simulink model "test_01"  (R2022b)
settings: Solver=VariableStepAuto  StartTime=0.0  StopTime=5  RelTol=1e-3
values from neighbouring files (symbols this model uses):
  C = Vout*(1-d/100)/(8*dV*f*f*L)    (= 6.25e-05)    [params.m]
  L = Vout*(1-d/100)/(f*dI)    (= 0.00990566037736)    [params.m]
undefined symbols (not defined in the file or in its folder): Ion, Lithium
libraries: spsThyristorLib x6, spsSeriesRLCBranchLib x3, spsVoltageMeasurementLib x3, spsCurrentMeasurementLib x2, spsGroundLib x1, spsThreePhaseProgrammableVoltageSourceLib x1, spsThreePhaseVIMeasurementLib x1, spsBatteryLib x1, spsDiodeLib x1, spsIGBTDiodeLib x1, slpidlib x1, spsTriangleGeneratorLib x1
settings Model: Creator=sanke  LastModifiedBy=sanke
settings SolverCC: ZeroCrossAlgorithm=Adaptive
settings DebuggingCC: IgnoredZcDiagnostic=none

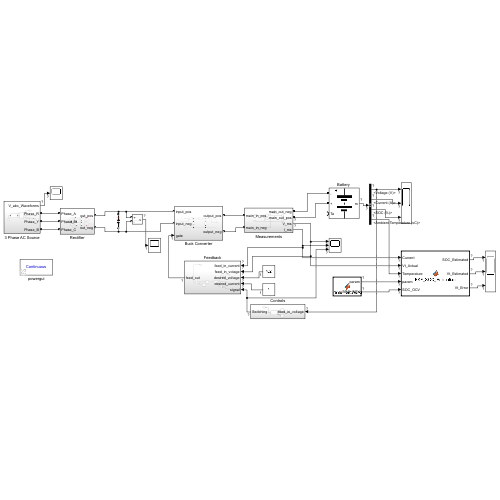
[thumbnail: Simulink's stored preview of the top-level diagram]
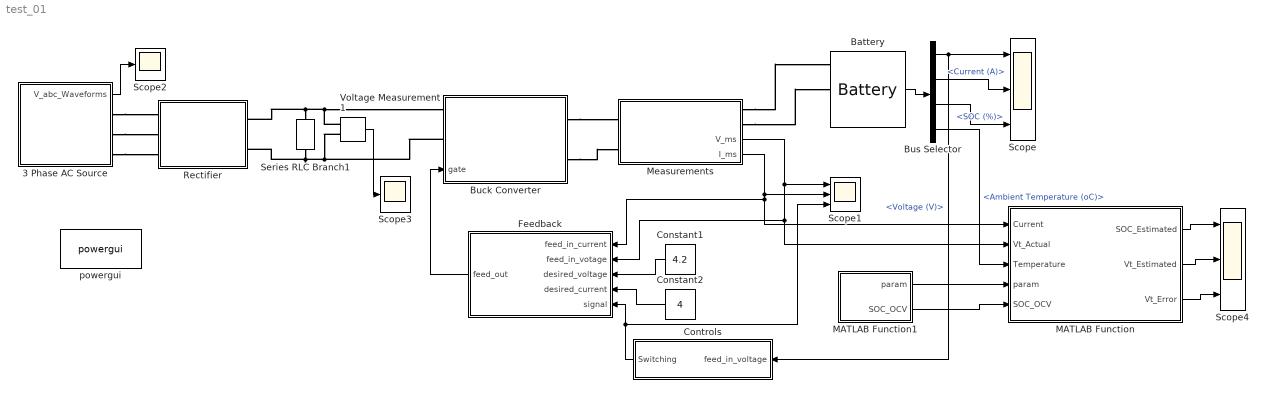
== system test_01 ==
  3 Phase AC Source : Subsystem
  "Battery " : spsBatteryLib/Battery  BatType=Lithium-Ion  ShowTempParam=on  ThermalPreset="3.6V  3.6Ah  (LiNiO2)"  ShowAgeParam=off  NomV=3.1  NomQ=3.6  SOC=55  Batt_Tr=30  PresetModel=off  MaxQ=3.2  MinV=2.325  FullV=3.75  Dis_rate=0.72  R=0.00889  Normal_OP=2.8  expZone="[3.5         0.5]"  current=[6.5 13 32.5]  Units=Time  Tci=20  NomT=20  T2=0  MaxQ2=2.7  FullV2=3.5  Normal_OP2=2.94  expZone2="[3.25         0.5]"  Rca=0.6  ti=1000  Dp=0  Neq0=0  Tsim=1e6  Ta1=25  Qeol=5.4*0.9  Reol=0.013333*1.2  Char_age=[2.3478, 3]  Dis_age=[2.3478, 10]  N1=1500  N2=10500  N3=1000  N4=1400  Ta2=45  N5=950
  Buck Converter : Subsystem
      settings: PortSchema="{\"entries\":[{\"content\":{\"sides\":[{\"content\":{\"connectorIds\":[\"LConn1\",\"LConn2\",\"In1\"]},\"type\":\"ConnectorPlacement.EquallySpacedRectSide\",\"uuid\":\"8046495b-0d90-4cb8-9891-48dc7aace6d4\"},{\"content\":{\"connectorIds\":[\"RConn1\",\"RConn2\"],\"side\":\"RIGHT\"},\"type\":\"ConnectorPlacement.EquallySpacedRectSide\",\"uuid\":\"421d384b-a39e-4e59-844e-5fb42b3432e4\"},{\"content\":{\"connectorIds\":[],\"side\":\"TOP\"},\"type\":\"ConnectorPlacement.EquallySpacedRectSide\",\"uuid\":\"a93954f5-8cef-4771-909c-d15532f662fe\"}]},\"type\":\"ConnectorPlacement.EquallySpacedConnector\",\"uuid\":\"185038a6-0d13-426c-9082-f1ae7959dda3\"}],\"packageUris\":[\"http://schema.mathworks.com/mf0/Connector/R2020b\"],\"version\":\"1.0\"}"
  Bus Selector : BusSelector  OutputSignals=Voltage (V),Current (A),SOC (%),Ambient Temperature (oC)
  Constant1 : Constant  Value=4.2
  Constant2 : Constant  Value=4
  Controls : Subsystem
  Feedback : Subsystem
  MATLAB Function : MATLAB Function  TreatAsAtomicUnit=on
  MATLAB Function1 : MATLAB Function  TreatAsAtomicUnit=on
  Measurements : Subsystem
      settings: PortSchema="{\"entries\":[{\"content\":{\"sides\":[{\"content\":{\"connectorIds\":[\"LConn1\",\"LConn2\"]},\"type\":\"ConnectorPlacement.EquallySpacedRectSide\",\"uuid\":\"fbcba962-5f19-4ca0-9e90-c21659520055\"},{\"content\":{\"connectorIds\":[\"RConn1\",\"RConn2\",\"Out1\",\"Out2\"],\"side\":\"RIGHT\"},\"type\":\"ConnectorPlacement.EquallySpacedRectSide\",\"uuid\":\"9e6fe38e-ff6b-4271-81f9-afd15cda60bb\"},{\"content\":{\"connectorIds\":[],\"side\":\"TOP\"},\"type\":\"ConnectorPlacement.EquallySpacedRectSide\",\"uuid\":\"0e1fc647-5705-4062-8d37-f05674e3ac40\"}]},\"type\":\"ConnectorPlacement.EquallySpacedConnector\",\"uuid\":\"9c5396ba-9d04-4277-89c0-94d7fbac7837\"}],\"packageUris\":[\"http://schema.mathworks.com/mf0/Connector/R2020b\"],\"version\":\"1.0\"}"
  Rectifier : Subsystem
  Scope : Scope  NumInputPorts=3
  Scope1 : Scope  NumInputPorts=3
  Scope2 : Scope
  Scope3 : Scope
  Scope4 : Scope  NumInputPorts=3
  Series RLC Branch1 : spsSeriesRLCBranchLib/Series RLC Branch  LConnTagsString=__new0  RConnTagsString=__new0  BranchType=C  Resistance=1  Inductance=1e-3  SetiL0=off  InitialCurrent=0  Capacitance=1000e-6  Setx0=off  InitialVoltage=0  Measurements=None
  Voltage Measurement1 : spsVoltageMeasurementLib/Voltage Measurement  PhasorSimulation=off  OutputType=Complex  PSBequivalent=0
  powergui : sps_lib/powergui  Priority=1  SimulationMode=Continuous  SampleTime=0.01  frequency=60  Iterations=50  frequencyindice=0  Pbase=100e6  ErrMax=1e-4  UnitsV=kV  UnitsW=MW  buscounter=0  FunctionMessages=off  echomessages=off  EnableUseOfTLC=off  CurrentSourceSwitches=off  DisableSnubberDevices=off  DisableRonSwitches=off  DisableVfSwitches=off  DisplayEquations=off  AutomaticDiscreteSolvers=off  SolverType=Tustin/Backward Euler (TBE)  Interpol=off  ExternalGateDelay=off  methode=off  Ts=100  x0status=blocks  SPID=on  SwTol=0  HookPort=off  NonlinearTolerance=1e-4  nMaxIteration=100  ContinueOnMaxIteration=off  RestoreLinks=warning  ResistiveCurrentMeasurement=off  Frange=[0:2:500]  Ylog=off  Xlog=on  ShowGrid=off  save=off  variable=ZData  structure=0  ZoomFFT=off  StartTime=0.0  cycles=1  DisplayStyle=1  fundamental=60  FreqAxis=off  MaxFrequency=1000  frequencyindicesteady=1  RmsSteady=1  display=off
  wires:
  Voltage Measurement1/1 -> Scope3/1
  3 Phase AC Source/1(V_abc_Waveforms) -> Scope2/1
  Constant1/1 -> Feedback/3(desired_voltage)
  Feedback/1(feed_out) -> Buck Converter/1(gate)
  Measurements/1(V_ms) -> MATLAB Function/2(Vt_Actual), Feedback/2(feed_in_votage), Scope1/1
  Measurements/2(I_ms) -> MATLAB Function/1(Current), Feedback/1(feed_in_current), Scope1/2
  Constant2/1 -> Feedback/4(desired_current)
  Controls/1(Switching) -> Scope1/3, Feedback/5(signal)
  "Battery "/1 -> Bus Selector/1
  Bus Selector/2 -> Scope/2  "<Current (A)>"
  Bus Selector/1 -> Controls/1(feed_in_voltage), Scope/1  "<Voltage (V)>"
  Bus Selector/3 -> Scope/3  "<SOC (%)>"
  Bus Selector/4 -> MATLAB Function/3(Temperature)  "<Ambient Temperature (oC)>"
  MATLAB Function/1(SOC_Estimated) -> Scope4/1
  MATLAB Function/2(Vt_Estimated) -> Scope4/2
  MATLAB Function/3(Vt_Error) -> Scope4/3
  MATLAB Function1/1(param) -> MATLAB Function/4(param)
  MATLAB Function1/2(SOC_OCV) -> MATLAB Function/5(SOC_OCV)
  connections:
  Voltage Measurement1/LConn1 -- Series RLC Branch1/LConn1 -- Rectifier/RConn1 -- Buck Converter/LConn1
  Voltage Measurement1/LConn2 -- Series RLC Branch1/RConn1 -- Rectifier/RConn2 -- Buck Converter/LConn2
  3 Phase AC Source/RConn1 -- Rectifier/LConn1
  3 Phase AC Source/RConn3 -- Rectifier/LConn3
  3 Phase AC Source/RConn2 -- Rectifier/LConn2
  Buck Converter/RConn2 -- Measurements/LConn2
  Buck Converter/RConn1 -- Measurements/LConn1
  Measurements/RConn1 -- "Battery "/LConn2
  Measurements/RConn2 -- "Battery "/LConn1

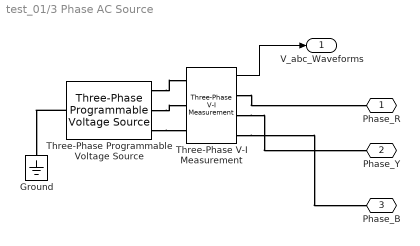
== system test_01/3 Phase AC Source ==
  Ground : spsGroundLib/Ground  LConnTagsString=a
  Three-Phase Programmable Voltage Source : spsThreePhaseProgrammableVoltageSourceLib/Three-Phase Programmable Voltage Source  PositiveSequence="[230*sqrt(2)  0 50]"  VariationEntity=None  VariationType=Table of time-amplitude pairs  VariationTypeAlt=Step  VariationStep=0.5  VariationRate=10  VariationMagnitude=0.3  VariationFrequency=2  VariationTiming=[1 2]  VariationPhaseA=off  Amplitudes=[1 0.8 1.2 1.0]  TimeValues=[0 0.1 0.15 0.2]  HarmonicGeneration=off  HarmonicA=[3 0.2 -25 0]  HarmonicB=[2 0.15 35 2]  Timing="[0.05  3]"  BusType=swing  Pref=0  Qref=0  Qmin=-inf  Qmax=inf
  Three-Phase V-I Measurement : spsThreePhaseVIMeasurementLib/Three-Phase V-I Measurement  VoltageMeasurement=phase-to-ground  SetLabelV=off  LabelV=Vabc  Vpu=off  VpuLL=off  CurrentMeasurement=no  SetLabelI=off  LabelI=Iabc  Ipu=off  Pbase=100e6  Vbase=500e3  OutputType=Complex  PhasorSimulation=off  PSBequivalent=0
  Phase_R : PMIOPort  Side=Right
  Phase_Y : PMIOPort  Port=2  Side=Right
  Phase_B : PMIOPort  Port=3  Side=Right
  V_abc_Waveforms : Outport
  wires:
  Three-Phase V-I Measurement/1 -> V_abc_Waveforms/1
  connections:
  Three-Phase Programmable Voltage Source/RConn1 -- Three-Phase V-I Measurement/LConn1
  Three-Phase Programmable Voltage Source/LConn1 -- Ground/LConn1
  Three-Phase Programmable Voltage Source/RConn2 -- Three-Phase V-I Measurement/LConn2
  Three-Phase Programmable Voltage Source/RConn3 -- Three-Phase V-I Measurement/LConn3
  Three-Phase V-I Measurement/RConn1 -- Phase_R/RConn1
  Three-Phase V-I Measurement/RConn2 -- Phase_Y/RConn1
  Three-Phase V-I Measurement/RConn3 -- Phase_B/RConn1

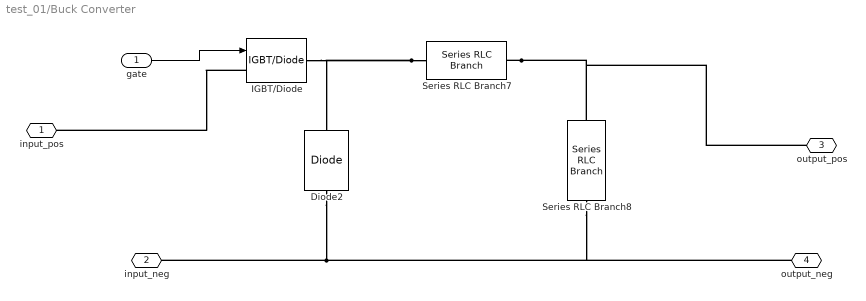
== system test_01/Buck Converter ==
  gate : Inport
  Diode2 : spsDiodeLib/Diode  Ron=0.001  Lon=0  Vf=0  IC=0  UseSnubber=0  Rs=500  Cs=250e-9  Measurements=off
  IGBT/Diode : spsIGBTDiodeLib/IGBT//Diode  Ron=1e-3  Rs=1e5  Cs=inf  Measurements=off
  Series RLC Branch7 : spsSeriesRLCBranchLib/Series RLC Branch  LConnTagsString=__new0  RConnTagsString=__new0  BranchType=L  Resistance=1  Inductance=L  SetiL0=off  InitialCurrent=0  Capacitance=1e-6  Setx0=off  InitialVoltage=0  Measurements=None
  Series RLC Branch8 : spsSeriesRLCBranchLib/Series RLC Branch  LConnTagsString=__new0  RConnTagsString=__new0  BranchType=C  Resistance=1  Inductance=1e-3  SetiL0=off  InitialCurrent=0  Capacitance=C  Setx0=off  InitialVoltage=0  Measurements=None
  input_pos : PMIOPort  Side=Left
  input_neg : PMIOPort  Port=2  Side=Left
  output_pos : PMIOPort  Port=3  Side=Right
  output_neg : PMIOPort  Port=4  Side=Right
  wires:
  gate/1 -> IGBT/Diode/1
  connections:
  IGBT/Diode/LConn1 -- input_pos/RConn1
  Series RLC Branch7/LConn1 -- IGBT/Diode/RConn1 -- Diode2/RConn1
  Series RLC Branch7/RConn1 -- output_pos/RConn1 -- Series RLC Branch8/LConn1
  Diode2/LConn1 -- Series RLC Branch8/RConn1 -- output_neg/RConn1 -- input_neg/RConn1

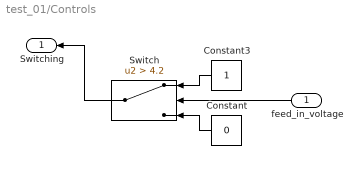
== system test_01/Controls ==
  feed_in_voltage : Inport
  Constant : Constant  Value=0
  Constant3 : Constant
  Switch : Switch  Criteria=u2 > Threshold  Threshold=4.2  SaturateOnIntegerOverflow=off  InputSameDT=off
  Switching : Outport
  wires:
  feed_in_voltage/1 -> Switch/2
  Switch/1 -> Switching/1
  Constant3/1 -> Switch/1
  Constant/1 -> Switch/3

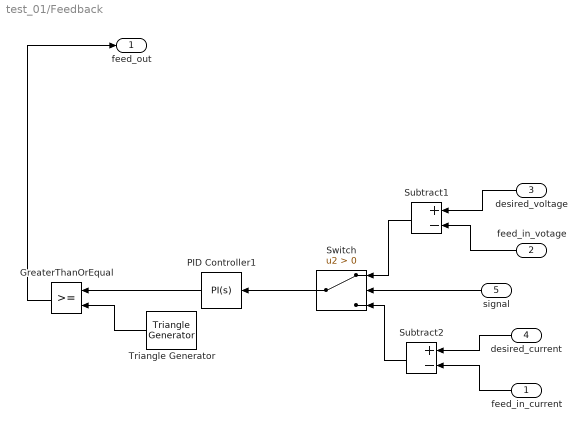
== system test_01/Feedback ==
  feed_in_current : Inport
  feed_in_votage : Inport  Port=2
  desired_voltage : Inport  Port=3
  desired_current : Inport  Port=4
  signal : Inport  Port=5
  GreaterThanOrEqual : RelationalOperator  OutDataTypeStr=boolean  RndMeth=Simplest  InputSameDT=off
  PID Controller1 : slpidlib/PID Controller  Controller=PI  Form=Parallel  TimeDomain=Continuous-time  UseExternalTs=off  SampleTime=-1  IntegratorMethod=Forward Euler  FilterMethod=Forward Euler  ControllerParametersSource=internal  P=50  I=5  UseKiTs=off  D=0  N=100  UseFilter=on  TunerSelectOption=Transfer Function Based (PID Tuner App)  InitialConditionSource=internal  InitialConditionForIntegrator=0  InitialConditionForFilter=0  DifferentiatorICPrevScaledInput=0  ExternalReset=none  TrackingMode=off  Kt=1  LimitOutput=off  SatLimitsSource=internal  UpperSaturationLimit=inf  LowerSaturationLimit=-inf  LinearizeAsGain=on  AntiWindupMode=none  Kb=1  LimitIntegrator=off  UpperIntegratorSaturationLimit=inf  LowerIntegratorSaturationLimit=-inf  POutMin=[]  POutMax=[]  IOutMin=[]  IOutMax=[]  DOutMin=[]  DOutMax=[]  NOutMin=[]  NOutMax=[]  SumOutMin=[]  SumOutMax=[]  SaturationOutMin=[]  SaturationOutMax=[]  PParamMin=[]  PParamMax=[]  IParamMin=[]  IParamMax=[]  DParamMin=[]  DParamMax=[]  NParamMin=[]  NParamMax=[]  KbParamMin=[]  KbParamMax=[]  KtParamMin=[]  KtParamMax=[]  KbOutMin=[]  KbOutMax=[]  KtOutMin=[]  KtOutMax=[]  IntegratorOutMin=[]  IntegratorOutMax=[]  FilterOutMin=[]  FilterOutMax=[]  SumI1OutMin=[]  SumI1OutMax=[]  SumI2OutMin=[]  SumI2OutMax=[]  SumI3OutMin=[]  SumI3OutMax=[]  SumI4OutMin=[]  SumI4OutMax=[]  SumDOutMin=[]  SumDOutMax=[]  DifferentiatorOutMin=[]  DifferentiatorOutMax=[]  FilterDiffOutCoefMin=[]  FilterDiffOutCoefMax=[]  ReciprocalOutMin=[]  ReciprocalOutMax=[]  SumDenOutMin=[]  SumDenOutMax=[]  SumNumOutMin=[]  SumNumOutMax=[]  DivideOutMin=[]  DivideOutMax=[]  UdiffTsProdOutMin=[]  UdiffTsProdOutMax=[]  NTsProdOutMin=[]  NTsProdOutMax=[]  UintegralTsProdOutMin=[]  UintegralTsProdOutMax=[]  UngainTsProdOutMin=[]  UngainTsProdOutMax=[]  ClampingZeroOutDataTypeStr=Inherit: Inherit via back propagation  ClampingZeroOutMin=[]  ClampingZeroOutMax=[]  FilterDenConstantOutDataTypeStr=Inherit: Inherit via back propagation  FilterDenConstantOutMin=[]  FilterDenConstantOutMax=[]  PCopyOutDataTypeStr=Inherit: Inherit via back propagation  PCopyOutMin=[]  PCopyOutMax=[]  NCopyOutDataTypeStr=Inherit: Inherit via back propagation  NCopyOutMin=[]  NCopyOutMax=[]  IntegratorContinuousStateAttributes=''  IntegratorStateMustResolveToSignalObject=off  IntegratorRTWStateStorageClass=Auto  FilterContinuousStateAttributes=''  FilterStateMustResolveToSignalObject=off  FilterRTWStateStorageClass=Auto  ParallelPVariant=InternalParameters  IdealPVariant=Disabled  IVariant=InternalParameters  DVariant=Disabled  IntegratorVariant=Continuous  SatVariant=Disabled  AWVariant=Passthrough  PCopyVariant=Disabled  TRVariant=Disabled  FdbkBlocksVariant=Forward  IdealPFdbkVariant=Disabled  SatFdbkVariant=Disabled  DerivativeFilterVariant=Disabled  NVariant=Disabled  NCopyVariant=Disabled_SignalSpec  FilterICVariant=Disabled  IntegratorICVariant=InternalICs  ExternalResetVariant=Disabled  TRSumVariant=Passthrough  SumFdbkVariant=Disabled  SumVariant=Sum_PI  TsampFilterVariant=InternalTs  TsampNgainVariant=Passthrough  TsampIntegralVariant=Passthrough  ExternalSaturationOutDataTypeStr=Inherit: Same as second input
  Subtract1 : Sum  Inputs=+-
  Subtract2 : Sum  Inputs=+-
  Switch : Switch  Criteria=u2 > Threshold  SaturateOnIntegerOverflow=off  InputSameDT=off
  Triangle Generator : spsTriangleGeneratorLib/Triangle Generator  Freq=25e3  Phase=90  Ts=0
  feed_out : Outport
  wires:
  Triangle Generator/1 -> GreaterThanOrEqual/2
  GreaterThanOrEqual/1 -> feed_out/1
  PID Controller1/1 -> GreaterThanOrEqual/1
  signal/1 -> Switch/2
  Subtract2/1 -> Switch/3
  desired_current/1 -> Subtract2/1
  feed_in_current/1 -> Subtract2/2
  desired_voltage/1 -> Subtract1/1
  feed_in_votage/1 -> Subtract1/2
  Subtract1/1 -> Switch/1
  Switch/1 -> PID Controller1/1

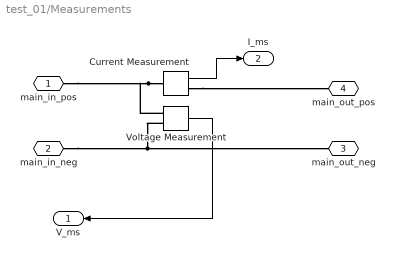
== system test_01/Measurements ==
  Current Measurement : spsCurrentMeasurementLib/Current Measurement  PhasorSimulation=off  OutputType=Complex  PSBequivalent=0
  Voltage Measurement : spsVoltageMeasurementLib/Voltage Measurement  PhasorSimulation=off  OutputType=Complex  PSBequivalent=0
  main_in_pos : PMIOPort  Side=Left
  main_in_neg : PMIOPort  Port=2  Side=Left
  main_out_neg : PMIOPort  Port=3  Side=Right
  main_out_pos : PMIOPort  Port=4  Side=Right
  V_ms : Outport
  I_ms : Outport  Port=2
  wires:
  Voltage Measurement/1 -> V_ms/1
  Current Measurement/1 -> I_ms/1
  connections:
  Current Measurement/LConn1 -- main_in_pos/RConn1 -- Voltage Measurement/LConn1
  Current Measurement/RConn1 -- main_out_pos/RConn1
  Voltage Measurement/LConn2 -- main_out_neg/RConn1 -- main_in_neg/RConn1

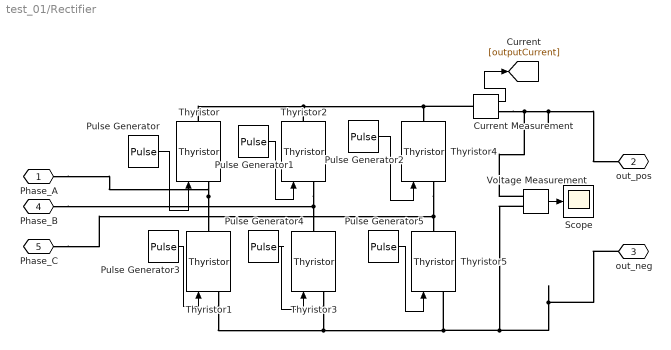
== system test_01/Rectifier ==
  Current Measurement : spsCurrentMeasurementLib/Current Measurement  PhasorSimulation=off  OutputType=Complex  PSBequivalent=0
  Pulse Generator : DiscretePulseGenerator  PulseType=Time based  Period=1/50  PulseWidth=33.33  PhaseDelay=(30+30)*0.02/360
  Pulse Generator1 : DiscretePulseGenerator  PulseType=Time based  Period=1/50  PulseWidth=33.33  PhaseDelay=(150+30)*0.02/360
  Pulse Generator2 : DiscretePulseGenerator  PulseType=Time based  Period=1/50  PulseWidth=33.33  PhaseDelay=(270+30)*0.02/360
  Pulse Generator3 : DiscretePulseGenerator  PulseType=Time based  Period=1/50  PulseWidth=33.33  PhaseDelay=(210+30)*0.02/360
  Pulse Generator4 : DiscretePulseGenerator  PulseType=Time based  Period=1/50  PulseWidth=33.33  PhaseDelay=(330+30)*0.02/360
  Pulse Generator5 : DiscretePulseGenerator  PulseType=Time based  Period=1/50  PulseWidth=33.33  PhaseDelay=(90+30)*0.02/360
  Scope : Scope
  Thyristor{,1..5} (6 alike) : spsThyristorLib/Thyristor  Ron=0.001  Lon=0  Vf=0.8  IC=0  Rs=500  Cs=250e-9  Measurements=off
  Voltage Measurement : spsVoltageMeasurementLib/Voltage Measurement  PhasorSimulation=off  OutputType=Complex  PSBequivalent=0
  Phase_A : PMIOPort  Side=Left
  out_pos : PMIOPort  Port=2  Side=Right
  out_neg : PMIOPort  Port=3  Side=Right
  Phase_B : PMIOPort  Port=4  Side=Left
  Phase_C : PMIOPort  Port=5  Side=Left
  wires:
  Pulse Generator2/1 -> Thyristor4/1
  Pulse Generator1/1 -> Thyristor2/1
  Current Measurement/1 -> [outputCurrent]
  Pulse Generator5/1 -> Thyristor5/1
  Pulse Generator/1 -> Thyristor/1
  Pulse Generator3/1 -> Thyristor1/1
  Pulse Generator4/1 -> Thyristor3/1
  Voltage Measurement/1 -> Scope/1
  connections:
  Thyristor/LConn1 -- Thyristor1/RConn1 -- Phase_A/RConn1
  Voltage Measurement/LConn1 -- Current Measurement/RConn1 -- out_pos/RConn1
  Thyristor/RConn1 -- Thyristor2/RConn1 -- Current Measurement/LConn1 -- Thyristor4/RConn1
  Thyristor1/LConn1 -- Thyristor3/LConn1 -- out_neg/RConn1 -- Voltage Measurement/LConn2 -- Thyristor5/LConn1
  Thyristor4/LConn1 -- Thyristor5/RConn1 -- Phase_C/RConn1
  Thyristor2/LConn1 -- Thyristor3/RConn1 -- Phase_B/RConn1

== matlab function test_01/MATLAB Function1 ==
  data: param output; SOC_OCV output
function [param, SOC_OCV] = getParamsFromWorkspace()
    % Fetch variables from the workspace
    param = evalin('base', 'param');
    SOC_OCV = evalin('base', 'SOC_OCV');
end

== matlab function test_01/MATLAB Function ==
  data: Current input; SOC_Estimated output; Vt_Actual input; Temperature input; Vt_Estimated output; Vt_Error output; param input; SOC_OCV input
function [SOC_Estimated, Vt_Estimated, Vt_Error] = EKF_SOC_Estimation(Current, Vt_Actual, Temperature, param, SOC_OCV)

SOC_Init    = 1; % intial SOC
X           = [SOC_Init; 0; 0]; % state space x parameter intializations
DeltaT      = 1; % sample time in seconds
Qn_rated    = 4.81 * 3600; % Ah to Amp-seconds

param = get_param(param);
SOC_OCV = get_param(SOC_OCV);

% initialize scatteredInterpolant functions for battery parameters and SOC-OCV curve
% this function also allows for extrapolation
F_R0    = scatteredInterpolant(param.T,param.SOC,param.R0);
F_R1    = scatteredInterpolant(param.T,param.SOC,param.R1);
F_R2    = scatteredInterpolant(param.T,param.SOC,param.R2);
F_C1    = scatteredInterpolant(param.T,param.SOC,param.C1);
F_C2    = scatteredInterpolant(param.T,param.SOC,param.C2);
% F_OCV   = scatteredInterpolant(param.T,param.SOC,param.OCV);  
% OCV can be extrapolated using the same method or through the polyfit function

SOCOCV  = polyfit(SOC_OCV.SOC,SOC_OCV.OCV,11); % calculate 11th order polynomial for the SOC-OCV curve 
dSOCOCV = polyder(SOCOCV); % derivative of SOC-OCV curve for matrix C

n_x   = size(X,1);
R_x   = 2.5e-5;
P_x   = [0.025 0 0;
         0 0.01 0;
         0 0 0.01];
Q_x   = [1.0e-6 0 0;
         0 1.0e-5 0;
         0 0 1.0e-5];

SOC_Estimated   = [];
Vt_Estimated    = [];
Vt_Error        = [];
ik              = length(Current);
% Current         = Current-0.1;

for k=1:1:ik
    T           = Temperature(k); % C
    U           = Current(k); % A
    SOC         = X(1);
    V1          = X(2);
    V2          = X(3);
    
    % Evaluate the battery parameter scatteredInterpolant 
    % functions for the current temperature & SOC
    R0     = F_R0(T,SOC);
    R1     = F_R1(T,SOC);
    R2     = F_R2(T,SOC);
    C1     = F_C1(T,SOC);
    C2     = F_C2(T,SOC);
    % OCV    = F_OCV(T,SOC);
    % OCV    = pchip(param.SOC,param.OCV,SOC); % pchip sample for unknown or single temperature
    
    OCV = polyval(SOCOCV,SOC); % calculate the values of OCV at the given SOC, using the polynomial SOCOCV
    Tau_1       = C1 * R1;
    Tau_2       = C2 * R2;
    
    a1 = exp(-DeltaT/Tau_1);
    a2 = exp(-DeltaT/Tau_2);
    
    b1 = R1 * (1 - exp(-DeltaT/Tau_1));
    b2 = R2 * (1 - exp(-DeltaT/Tau_2));
    TerminalVoltage = OCV - R0*U - V1 - V2;
    if U > 0
        eta = 1; % eta for discharging
    elseif U <= 0 
        eta = 1; % eta for charging
    end
    dOCV = polyval(dSOCOCV, SOC);
    C_x    = [dOCV -1 -1];
    Error_x   = Vt_Actual(k) - TerminalVoltage;
    Vt_Estimated    = [Vt_Estimated;TerminalVoltage];
    SOC_Estimated   = [SOC_Estimated;X(1)];
    Vt_Error        = [Vt_Error;Error_x];
    A   = [1 0  0;
           0 a1 0;
           0 0  a2];
    B   = [-(eta * DeltaT/Qn_rated); b1; b2];
    X   = (A * X) + (B * U);
    P_x = (A * P_x * A') + Q_x;
    KalmanGain_x = (P_x) * (C_x') * (inv((C_x * P_x * C_x') + (R_x)));
    X            = X + (KalmanGain_x * Error_x);
    P_x          = (eye(n_x,n_x) - (KalmanGain_x * C_x)) * P_x;

end
